simulink model "Droopslx"  (R2021a)
settings: Solver=FixedStepDiscrete  StartTime=0.0  StopTime=0.3  FixedStep=1e-6  RelTol=1e-3
InitFcn:
  | %%Elec
  | Vdc=400;
  | L=1.2e-3;
  | Cf=1e-6;
  | R_Load=20;
  | R1=0.005;
  | 
  | %%PWM
  | f=20000;
  | Ts=1/f;
  | w=314.15926;
  | 
  | %%PID
  | Kpi=30;
  | Kpu=0.1;
  | Kiu=600;
  | 
  | %%下垂控制
  | Ksogi=1;
  | m=0.00038;
  | n=0.001;
  | w_lp=2*pi*25;
  | wref=314.15926;
  | Lv=1e-3;
  | 
  | t1=0.14;
  | t2=0.14;
undefined symbols (not defined in the file): DiscIntNeverNeededParam
libraries: spsSeriesRLCBranchLib x15, spsIGBTDiodeLib x8, simulink x4, spsMultimeterLib x4, spsVoltageMeasurementLib x4, spsBreakerLib x3, spsDCVoltageSourceLib x2, pid_lib x2, spsAlphaBetaZerotodq0Lib x1, spspowerguiLib x1
settings Model: Creator=45276  LastModifiedBy=45276
settings DebuggingCC: UnconnectedInputMsg=none  UnconnectedOutputMsg=none  UnconnectedLineMsg=none

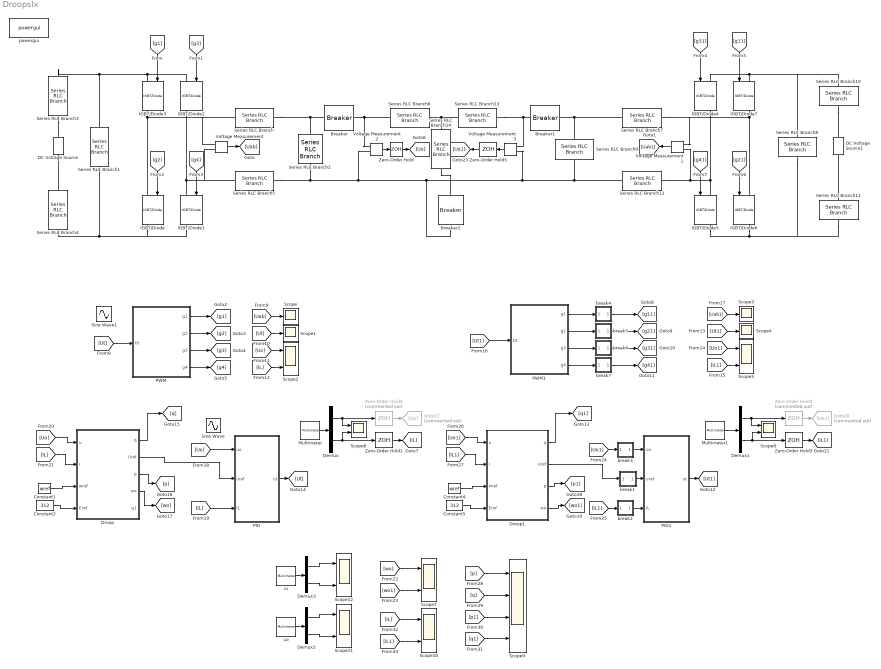
== system Droopslx ==
  Breaker : spsBreakerLib/Breaker  InitialState=0  SwitchingTimes=0  External=off  BreakerResistance=0.0001  SnubberResistance=1e6  SnubberCapacitance=inf  Measurements=None  MoreParameters=on  NoBreakLoop=off
      settings: SourceProductBaseCode=PS
  Breaker1 : spsBreakerLib/Breaker  InitialState=0  SwitchingTimes=t2  External=off  BreakerResistance=0.0001  SnubberResistance=1e6  SnubberCapacitance=inf  Measurements=None  MoreParameters=on  NoBreakLoop=off
      settings: SourceProductBaseCode=PS
  Breaker2 : spsBreakerLib/Breaker  InitialState=0  SwitchingTimes=0.0  External=off  BreakerResistance=0.0001  SnubberResistance=1e6  SnubberCapacitance=inf  Measurements=None  MoreParameters=on  NoBreakLoop=off
      settings: SourceProductBaseCode=PS
  Constant1 : Constant  Value=wref
  Constant2 : Constant  Value=312
  Constant4 : Constant  Value=wref
  Constant5 : Constant  Value=312
  DC Voltage Source : spsDCVoltageSourceLib/DC Voltage Source  Amplitude=Vdc  Measurements=None
  DC Voltage Source1 : spsDCVoltageSourceLib/DC Voltage Source  Amplitude=Vdc  Measurements=None
  Demux{,1..3} (4 alike) : Demux  Outputs=2
  Droop : Subsystem
  Droop1 : Subsystem
  Goto20 : Goto  Commented=on  GotoTag=Uo1
  Goto22 : Goto  Commented=on  GotoTag=Uo
  IGBT/Diode{,1..7} (8 alike) : spsIGBTDiodeLib/IGBT//Diode  Ron=1e-3  Rs=1e5  Cs=inf  Measurements=on
  Multimeter : spsMultimeterLib/Multimeter  PhasorSimulation=off  OutputType=Complex  sel=[1 4]  L=7  Gain=[1 1]  yselected={'Ub: Series RLC Branch2','Ib: Series RLC Branch'};  PSBOutputType=1  PSBequivalent=0  AxesSetting=[0,0.1,-100,100]  Display=0  SavedBlockNames=-11
  Multimeter1 : spsMultimeterLib/Multimeter  PhasorSimulation=off  OutputType=Complex  sel=[3 7]  L=7  Gain=[1 1]  yselected={'Ub: Series RLC Branch9','Ib: Series RLC Branch7'};  PSBOutputType=1  PSBequivalent=0  AxesSetting=[0,0.1,-100,100]  Display=0  SavedBlockNames=-11
  PID : Subsystem
  PID1 : Subsystem
  PWM : Subsystem
  PWM1 : Subsystem
  Scope{,1,3..4} (4 alike) : Scope
  Scope{2,5..8,10..12} (8 alike) : Scope  NumInputPorts=2
  Scope9 : Scope  NumInputPorts=4
  Series RLC Branch : spsSeriesRLCBranchLib/Series RLC Branch  LConnTagsString=__new0  RConnTagsString=__new0  BranchType=RL  Resistance=R1/2  Inductance=L  SetiL0=off  InitialCurrent=0  Capacitance=1e-6  Setx0=off  InitialVoltage=0  Measurements=Branch current
  Series RLC Branch1 : spsSeriesRLCBranchLib/Series RLC Branch  LConnTagsString=__new0  RConnTagsString=__new0  BranchType=C  Resistance=1  Inductance=1e-3  SetiL0=off  InitialCurrent=0  Capacitance=Cf  Setx0=off  InitialVoltage=0  Measurements=None
  Series RLC Branch{3..4,10..11} (4 alike) : spsSeriesRLCBranchLib/Series RLC Branch  LConnTagsString=__new0  RConnTagsString=__new0  BranchType=R  Resistance=R1  Inductance=1e-3  SetiL0=off  InitialCurrent=0  Capacitance=1e-6  Setx0=off  InitialVoltage=0  Measurements=None
  Series RLC Branch12 : spsSeriesRLCBranchLib/Series RLC Branch  LConnTagsString=__new0  RConnTagsString=__new0  BranchType=RL  Resistance=R1/2  Inductance=L  SetiL0=off  InitialCurrent=0  Capacitance=1e-6  Setx0=off  InitialVoltage=0  Measurements=None
  Series RLC Branch13 : spsSeriesRLCBranchLib/Series RLC Branch  LConnTagsString=__new0  RConnTagsString=__new0  BranchType=R  Resistance=0.005  Inductance=1e-3  SetiL0=off  InitialCurrent=0  Capacitance=1e-6  Setx0=off  InitialVoltage=0  Measurements=Branch current
  Series RLC Branch14 : spsSeriesRLCBranchLib/Series RLC Branch  LConnTagsString=__new0  RConnTagsString=__new0  BranchType=R  Resistance=R_Load  Inductance=1e-3  SetiL0=off  InitialCurrent=0  Capacitance=1e-6  Setx0=off  InitialVoltage=0  Measurements=None
  Series RLC Branch2 : spsSeriesRLCBranchLib/Series RLC Branch  LConnTagsString=__new0  RConnTagsString=__new0  BranchType=C  Resistance=1  Inductance=1e-3  SetiL0=off  InitialCurrent=0  Capacitance=Cf  Setx0=off  InitialVoltage=0  Measurements=Branch voltage
  Series RLC Branch5 : spsSeriesRLCBranchLib/Series RLC Branch  LConnTagsString=__new0  RConnTagsString=__new0  BranchType=RL  Resistance=R1/2  Inductance=L  SetiL0=off  InitialCurrent=0  Capacitance=1e-6  Setx0=off  InitialVoltage=0  Measurements=None
  Series RLC Branch6 : spsSeriesRLCBranchLib/Series RLC Branch  LConnTagsString=__new0  RConnTagsString=__new0  BranchType=R  Resistance=0.001  Inductance=1e-3  SetiL0=off  InitialCurrent=0  Capacitance=1e-6  Setx0=off  InitialVoltage=0  Measurements=Branch voltage and current
  Series RLC Branch7 : spsSeriesRLCBranchLib/Series RLC Branch  LConnTagsString=__new0  RConnTagsString=__new0  BranchType=RL  Resistance=R1/2  Inductance=L  SetiL0=off  InitialCurrent=0  Capacitance=1e-6  Setx0=off  InitialVoltage=0  Measurements=Branch current
  Series RLC Branch8 : spsSeriesRLCBranchLib/Series RLC Branch  LConnTagsString=__new0  RConnTagsString=__new0  BranchType=C  Resistance=1  Inductance=1e-3  SetiL0=off  InitialCurrent=0  Capacitance=Cf  Setx0=off  InitialVoltage=0  Measurements=None
  Series RLC Branch9 : spsSeriesRLCBranchLib/Series RLC Branch  LConnTagsString=__new0  RConnTagsString=__new0  BranchType=C  Resistance=1  Inductance=1e-3  SetiL0=off  InitialCurrent=0  Capacitance=Cf  Setx0=off  InitialVoltage=0  Measurements=Branch voltage
  Sine Wave : Sin  Amplitude=400  Frequency=2*pi*50  SampleTime=Ts
  Sine Wave1 : Sin  Frequency=2*pi*50  SampleTime=0
  Voltage Measurement{,1..3} (4 alike) : spsVoltageMeasurementLib/Voltage Measurement  PhasorSimulation=off  OutputType=Complex  PSBequivalent=0
  Zero-Order Hold : ZeroOrderHold  SampleTime=Ts
  Zero-Order Hold1 : ZeroOrderHold  SampleTime=Ts
  Zero-Order Hold2 : ZeroOrderHold  Commented=on  SampleTime=-1
  Zero-Order Hold3 : ZeroOrderHold  SampleTime=-1
  Zero-Order Hold4 : ZeroOrderHold  Commented=on  SampleTime=Ts
  Zero-Order Hold5 : ZeroOrderHold  SampleTime=Ts
  break1 : Subsystem
  break2 : Subsystem
  break3 : Subsystem
  break4 : Subsystem
  break5 : Subsystem
  break6 : Subsystem
  break7 : Subsystem
  io : spsMultimeterLib/Multimeter  PhasorSimulation=off  OutputType=Complex  sel=[6 5]  L=7  Gain=[1 1]  yselected={'Ib: Series RLC Branch6','Ib: Series RLC Branch13'};  PSBOutputType=1  PSBequivalent=0  AxesSetting=[0,0.1,-100,100]  Display=0  SavedBlockNames=-11
  powergui : spspowerguiLib/powergui  Priority=1  SimulationMode=Discrete  SampleTime=1e-6  frequency=60  Iterations=50  frequencyindice=0  Pbase=100e6  ErrMax=1e-4  UnitsV=kV  UnitsW=MW  buscounter=0  FunctionMessages=off  echomessages=off  EnableUseOfTLC=off  CurrentSourceSwitches=off  DisableSnubberDevices=off  DisableRonSwitches=off  DisableVfSwitches=off  DisplayEquations=off  AutomaticDiscreteSolvers=off  SolverType=Tustin/Backward Euler (TBE)  Interpol=off  ExternalGateDelay=off  methode=off  Ts=100  x0status=blocks  SPID=on  SwTol=0  HookPort=off  NonlinearTolerance=1e-4  nMaxIteration=100  ContinueOnMaxIteration=off  RestoreLinks=warning  ResistiveCurrentMeasurement=off  Frange=[0:2:500]  Ylog=off  Xlog=on  ShowGrid=off  save=off  variable=ZData  structure=0  ZoomFFT=off  StartTime=0.0  cycles=1  DisplayStyle=1  fundamental=60  FreqAxis=off  MaxFrequency=1000  frequencyindicesteady=1  RmsSteady=1  display=off
  uo : spsMultimeterLib/Multimeter  PhasorSimulation=off  OutputType=Complex  sel=[1 3]  L=7  Gain=[1 1]  yselected={'Ub: Series RLC Branch2','Ub: Series RLC Branch9'};  PSBOutputType=1  PSBequivalent=0  AxesSetting=[0,0.1,-100,100]  Display=0  SavedBlockNames=-11
  wires:
  Voltage Measurement/1 -> [Uab]
  Voltage Measurement1/1 -> [Uab1]
  [g1] -> IGBT/Diode3/1
  [g3] -> IGBT/Diode2/1
  [g4] -> IGBT/Diode1/1
  [g2] -> IGBT/Diode/1
  [g31] -> IGBT/Diode4/1
  [g11] -> IGBT/Diode7/1
  [g41] -> IGBT/Diode5/1
  [g21] -> IGBT/Diode6/1
  PWM/1(g1) -> [g1]
  PWM/2(g2) -> [g2]
  PWM/3(g3) -> [g3]
  PWM/4(g4) -> [g4]
  [Uab] -> Scope/1
  [Ut] -> Scope1/1
  [Uo] -> Scope2/1
  [IL] -> Scope2/2
  [IL1] -> Scope5/2
  [Uo1] -> Scope5/1
  [Ut1] -> Scope4/1
  [Uab1] -> Scope3/1
  PWM1/1(g1) -> break4/1(in)
  [Ut1] -> PWM1/1(Ut)
  [IL] -> PID/3(IL)
  PID/1(ut) -> [Ut]
  [Uo] -> Droop/1(u)
  Constant1/1 -> Droop/3(wref)
  Constant2/1 -> Droop/4(Eref)
  Droop/1(q) -> [q]
  Droop/3(p) -> [p]
  Droop/4(wo) -> [wo]
  Multimeter/1 -> Demux/1
  Demux/2 -> Scope6/2, Zero-Order Hold1/1
  Demux/1 -> Zero-Order Hold4/1, Scope6/1
  Zero-Order Hold1/1 -> [IL]
  [wo] -> Scope7/1
  [wo1] -> Scope7/2
  Zero-Order Hold3/1 -> [IL1]
  Zero-Order Hold2/1 -> Goto20/1
  Demux1/1 -> Zero-Order Hold2/1, Scope8/1
  Demux1/2 -> Zero-Order Hold3/1, Scope8/2
  Multimeter1/1 -> Demux1/1
  Droop1/4(wo) -> [wo1]
  Droop1/3(p) -> [p1]
  Droop1/1(q) -> [q1]
  Constant5/1 -> Droop1/4(Eref)
  Constant4/1 -> Droop1/3(wref)
  [Uo1] -> Droop1/1(u)
  PID1/1(ut) -> [Ut1]
  [IL1] -> break2/1(in)
  [p] -> Scope9/1
  [q] -> Scope9/2
  [p1] -> Scope9/3
  [q1] -> Scope9/4
  [IL1] -> Droop1/2(I)
  [Uo] -> PID/1(uo)
  [Uo1] -> break3/1(in)
  [Ut] -> PWM/1(Ut)
  Droop/2(Uref) -> PID/2(uref)
  [IL] -> Droop/2(I)
  [IL] -> Scope10/1
  [IL1] -> Scope10/2
  break2/1(out) -> PID1/3(IL)
  break3/1(out) -> PID1/1(uo)
  Droop1/2(Uref) -> break1/1(in)
  break4/1(out) -> [g11]
  PWM1/2(g2) -> break5/1(in)
  break5/1(out) -> [g21]
  PWM1/3(g3) -> break6/1(in)
  break6/1(out) -> [g31]
  PWM1/4(g4) -> break7/1(in)
  break7/1(out) -> [g41]
  Zero-Order Hold/1 -> [Uo]
  Voltage Measurement2/1 -> Zero-Order Hold/1
  Zero-Order Hold4/1 -> Goto22/1
  Zero-Order Hold5/1 -> [Uo1]
  Voltage Measurement3/1 -> Zero-Order Hold5/1
  break1/1(out) -> PID1/2(uref)
  Demux2/1 -> Scope11/1
  Demux2/2 -> Scope11/2
  uo/1 -> Demux2/1
  io/1 -> Demux3/1
  Demux3/1 -> Scope12/1
  Demux3/2 -> Scope12/2
  connections:
  Series RLC Branch4/LConn1 -- DC Voltage Source/LConn1
  Series RLC Branch3/RConn1 -- DC Voltage Source/RConn1
  Series RLC Branch3/LConn1 -- Series RLC Branch1/LConn1 -- IGBT/Diode3/LConn1 -- IGBT/Diode2/LConn1
  Voltage Measurement/LConn1 -- Series RLC Branch/LConn1 -- IGBT/Diode3/RConn1 -- IGBT/Diode/LConn1
  IGBT/Diode1/RConn1 -- IGBT/Diode/RConn1 -- Series RLC Branch1/RConn1 -- Series RLC Branch4/RConn1
  Voltage Measurement/LConn2 -- Series RLC Branch5/LConn1 -- IGBT/Diode2/RConn1 -- IGBT/Diode1/LConn1
  Series RLC Branch/RConn1 -- Breaker/LConn1 -- Series RLC Branch2/LConn1
  Series RLC Branch8/LConn1 -- Series RLC Branch10/LConn1 -- IGBT/Diode7/LConn1 -- IGBT/Diode4/LConn1
  Voltage Measurement1/LConn2 -- Series RLC Branch7/LConn1 -- IGBT/Diode7/RConn1 -- IGBT/Diode6/LConn1
  Series RLC Branch11/RConn1 -- Series RLC Branch8/RConn1 -- IGBT/Diode6/RConn1 -- IGBT/Diode5/RConn1
  Series RLC Branch12/LConn1 -- Voltage Measurement1/LConn1 -- IGBT/Diode5/LConn1 -- IGBT/Diode4/RConn1
  Series RLC Branch7/RConn1 -- Breaker1/RConn1 -- Series RLC Branch9/LConn1
  Series RLC Branch12/RConn1 -- Voltage Measurement3/LConn2 -- Breaker2/LConn1 -- Voltage Measurement2/LConn2 -- Series RLC Branch5/RConn1 -- Series RLC Branch2/RConn1 -- Series RLC Branch9/RConn1
  Series RLC Branch11/LConn1 -- DC Voltage Source1/LConn1
  Series RLC Branch10/RConn1 -- DC Voltage Source1/RConn1
  Series RLC Branch6/LConn1 -- Series RLC Branch14/LConn1 -- Series RLC Branch13/LConn1
  Series RLC Branch13/RConn1 -- Voltage Measurement3/LConn1 -- Breaker1/LConn1
  Breaker/RConn1 -- Voltage Measurement2/LConn1 -- Series RLC Branch6/RConn1
  Series RLC Branch14/RConn1 -- Breaker2/RConn1

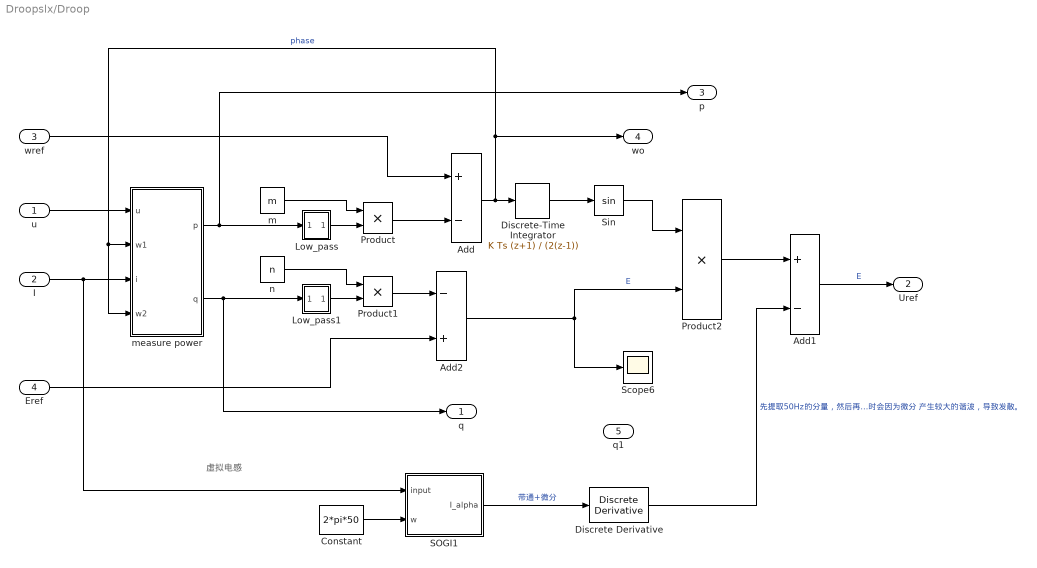
== system Droopslx/Droop ==
  note: 虚拟电感
  u : Inport
  I : Inport  Port=2
  wref : Inport  Port=3
  Eref : Inport  Port=4
  Add : Sum  Inputs=+-
  Add1 : Sum  Inputs=+-
  Add2 : Sum  Inputs=-+
  Constant : Constant  Value=2*pi*50
  Discrete Derivative : simulink/Discrete/Discrete Derivative  gainval=Lv  ICPrevScaledInput=0.0  OutMin=[]  OutMax=[]  OutDataType=fixdt(1, 16)  OutScaling=2^-10  DoSatur=off
  Discrete-Time Integrator : DiscreteIntegrator  IntegratorMethod=Integration: Trapezoidal  SampleTime=Ts  ICPrevOutput=DiscIntNeverNeededParam  ICPrevScaledInput=DiscIntNeverNeededParam
  Low_pass : Subsystem
  Low_pass1 : Subsystem
  Product : Product
  Product1 : Product
  Product2 : Product
  SOGI1 : Subsystem
  Scope6 : Scope
  Sin : Trigonometry
  m : Constant  Value=m
  measure power : Subsystem
  n : Constant  Value=n
  q : Outport
  Uref : Outport  Port=2
  p : Outport  Port=3
  wo : Outport  Port=4
  q1 : Outport  Port=5
  wires:
  measure power/1(p) -> p/1, Low_pass/1(in)
  Add2/1 -> Scope6/1, Product2/2  "E"
  Add/1 -> measure power/4(w2), measure power/2(w1), wo/1, Discrete-Time Integrator/1  "phase"
  measure power/2(q) -> q/1, Low_pass1/1(in)
  Discrete-Time Integrator/1 -> Sin/1
  I/1 -> SOGI1/1(input), measure power/3(i)
  m/1 -> Product/1
  Product2/1 -> Add1/1
  Low_pass/1(out) -> Product/2
  Sin/1 -> Product2/1
  Product1/1 -> Add2/1
  n/1 -> Product1/1
  Eref/1 -> Add2/2
  u/1 -> measure power/1(u)
  Low_pass1/1(out) -> Product1/2
  Add1/1 -> Uref/1  "E"
  Product/1 -> Add/2
  wref/1 -> Add/1
  SOGI1/1(I_alpha) -> Discrete Derivative/1  "带通+微分"
  Constant/1 -> SOGI1/2(w)
  Discrete Derivative/1 -> Add1/2  "先提取50Hz的分量，然后再取微分。 如果先取微分，再用SOGI提取时会因为微分 产生较大的谐波，导致发散。"

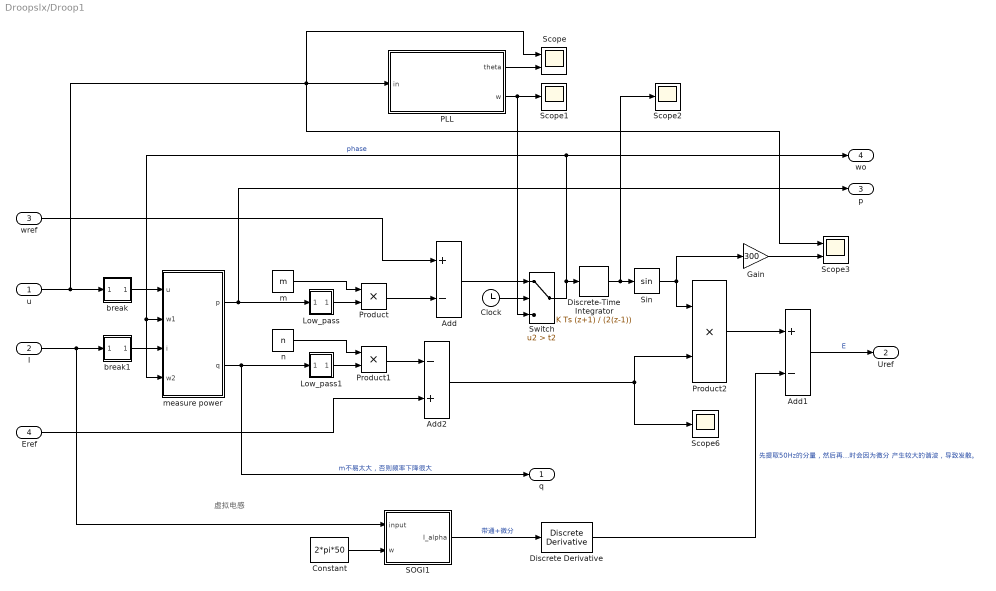
== system Droopslx/Droop1 ==
  note: 虚拟电感
  u : Inport
  I : Inport  Port=2
  wref : Inport  Port=3
  Eref : Inport  Port=4
  Add : Sum  Inputs=+-
  Add1 : Sum  Inputs=+-
  Add2 : Sum  Inputs=-+
  Clock : Clock
  Constant : Constant  Value=2*pi*50
  Discrete Derivative : simulink/Discrete/Discrete Derivative  gainval=Lv  ICPrevScaledInput=0.0  OutMin=[]  OutMax=[]  OutDataType=fixdt(1, 16)  OutScaling=2^-10  DoSatur=off
  Discrete-Time Integrator : DiscreteIntegrator  IntegratorMethod=Integration: Trapezoidal  SampleTime=Ts  ICPrevOutput=DiscIntNeverNeededParam  ICPrevScaledInput=DiscIntNeverNeededParam
  Gain : Gain  Gain=300
  Low_pass : Subsystem
  Low_pass1 : Subsystem
  PLL : Subsystem
  Product : Product
  Product1 : Product
  Product2 : Product
  SOGI1 : Subsystem
  Scope : Scope  NumInputPorts=2
  Scope1 : Scope
  Scope2 : Scope
  Scope3 : Scope  NumInputPorts=2
  Scope6 : Scope
  Sin : Trigonometry
  Switch : Switch  Criteria=u2 > Threshold  Threshold=t2
  break : Subsystem
  break1 : Subsystem
  m : Constant  Value=m
  measure power : Subsystem
  n : Constant  Value=n
  q : Outport
  Uref : Outport  Port=2
  p : Outport  Port=3
  wo : Outport  Port=4
  wires:
  wref/1 -> Add/1
  Product/1 -> Add/2
  Add1/1 -> Uref/1  "E"
  Low_pass1/1(out) -> Product1/2
  u/1 -> break/1(in), Scope3/1, Scope/1, PLL/1(in)
  Eref/1 -> Add2/2
  n/1 -> Product1/1
  Product1/1 -> Add2/1
  Sin/1 -> Product2/1, Gain/1
  Low_pass/1(out) -> Product/2
  Product2/1 -> Add1/1
  m/1 -> Product/1
  I/1 -> SOGI1/1(input), break1/1(in)
  Discrete-Time Integrator/1 -> Scope2/1, Sin/1
  measure power/2(q) -> Low_pass1/1(in), q/1  "m不易太大，否则频率下降很大"
  Add/1 -> Switch/1
  Add2/1 -> Product2/2, Scope6/1
  measure power/1(p) -> Low_pass/1(in), p/1
  Clock/1 -> Switch/2
  Switch/1 -> wo/1, measure power/4(w2), measure power/2(w1), Discrete-Time Integrator/1  "phase"
  Gain/1 -> Scope3/2
  PLL/1(theta) -> Scope/2
  PLL/2(w) -> Switch/3, Scope1/1
  break/1(out) -> measure power/1(u)
  break1/1(out) -> measure power/3(i)
  Constant/1 -> SOGI1/2(w)
  SOGI1/1(I_alpha) -> Discrete Derivative/1  "带通+微分"
  Discrete Derivative/1 -> Add1/2  "先提取50Hz的分量，然后再取微分。 如果先取微分，再用SOGI提取时会因为微分 产生较大的谐波，导致发散。"

== system Droopslx/PID ==
  note: 前馈控制
  note: 电压环
  note: 电流环
  uo : Inport
  uref : Inport  Port=2
  IL : Inport  Port=3
  Gain : Gain  Gain=Kpi
  Gain1 : Gain  Gain=1/400
  PID Controller : pid_lib/PID Controller  Controller=PI  Form=Parallel  TimeDomain=Discrete-time  UseExternalTs=off  SampleTime=Ts  IntegratorMethod=Trapezoidal  FilterMethod=Forward Euler  ControllerParametersSource=internal  P=Kpu  I=Kiu  D=0  UseFilter=on  N=100  TunerSelectOption=Transfer Function Based (PID Tuner App)  InitialConditionSource=internal  InitialConditionForIntegrator=0  InitialConditionForFilter=0  DifferentiatorICPrevScaledInput=0  ExternalReset=none  TrackingMode=off  Kt=1  LimitOutput=off  SatLimitsSource=internal  UpperSaturationLimit=inf  LowerSaturationLimit=-inf  LinearizeAsGain=on  AntiWindupMode=none  Kb=1  POutMin=[]  POutMax=[]  IOutMin=[]  IOutMax=[]  DOutMin=[]  DOutMax=[]  NOutMin=[]  NOutMax=[]  SumOutMin=[]  SumOutMax=[]  SaturationOutMin=[]  SaturationOutMax=[]  PParamMin=[]  PParamMax=[]  IParamMin=[]  IParamMax=[]  DParamMin=[]  DParamMax=[]  NParamMin=[]  NParamMax=[]  KbParamMin=[]  KbParamMax=[]  KtParamMin=[]  KtParamMax=[]  KbOutMin=[]  KbOutMax=[]  KtOutMin=[]  KtOutMax=[]  IntegratorOutMin=[]  IntegratorOutMax=[]  FilterOutMin=[]  FilterOutMax=[]  SumI1OutMin=[]  SumI1OutMax=[]  SumI2OutMin=[]  SumI2OutMax=[]  SumI3OutMin=[]  SumI3OutMax=[]  SumI4OutMin=[]  SumI4OutMax=[]  SumDOutMin=[]  SumDOutMax=[]  DifferentiatorOutMin=[]  DifferentiatorOutMax=[]  FilterDiffOutCoefMin=[]  FilterDiffOutCoefMax=[]  ReciprocalOutMin=[]  ReciprocalOutMax=[]  SumDenOutMin=[]  SumDenOutMax=[]  SumNumOutMin=[]  SumNumOutMax=[]  DivideOutMin=[]  DivideOutMax=[]  UdiffTsProdOutMin=[]  UdiffTsProdOutMax=[]  NTsProdOutMin=[]  NTsProdOutMax=[]  UintegralTsProdOutMin=[]  UintegralTsProdOutMax=[]  UngainTsProdOutMin=[]  UngainTsProdOutMax=[]  IntegratorContinuousStateAttributes=''  IntegratorStateMustResolveToSignalObject=off  IntegratorRTWStateStorageClass=Auto  FilterContinuousStateAttributes=''  FilterStateMustResolveToSignalObject=off  FilterRTWStateStorageClass=Auto  ParallelPVariant=InternalParameters  IdealPVariant=Disabled  IVariant=InternalParameters  DVariant=Disabled  IntegratorVariant=Discrete  SatVariant=Disabled  AWVariant=Passthrough  PCopyVariant=Disabled  TRVariant=Disabled  FdbkBlocksVariant=Forward  IdealPFdbkVariant=Disabled  SatFdbkVariant=Disabled  DerivativeFilterVariant=Disabled  NVariant=Disabled  NCopyVariant=Disabled_SignalSpec  FilterICVariant=Disabled  IntegratorICVariant=InternalICs  ExternalResetVariant=Disabled  TRSumVariant=Passthrough  SumFdbkVariant=Disabled  SumVariant=Sum_PI  TsampFilterVariant=InternalTs  TsampNgainVariant=Passthrough  TsampIntegralVariant=Passthrough  ExternalSaturationOutDataTypeStr=Inherit: Same as second input
  Sum : Sum  Inputs=|+-
  Sum1 : Sum  Inputs=|+-
  Sum2 : Sum  Inputs=|++
  ut : Outport
  wires:
  Gain/1 -> Sum2/1
  PID Controller/1 -> Sum1/1
  Sum1/1 -> Gain/1
  uo/1 -> Sum2/2, Sum/2
  IL/1 -> Sum1/2
  uref/1 -> Sum/1
  Sum/1 -> PID Controller/1
  Sum2/1 -> Gain1/1
  Gain1/1 -> ut/1

== system Droopslx/PID1 ==
  note: 电流环
  note: 电压环
  uo : Inport
  uref : Inport  Port=2
  IL : Inport  Port=3
  Gain : Gain  Gain=Kpi
  Gain1 : Gain  Gain=1/400
  PID Controller : pid_lib/PID Controller  Controller=PI  Form=Parallel  TimeDomain=Discrete-time  UseExternalTs=off  SampleTime=Ts  IntegratorMethod=Trapezoidal  FilterMethod=Forward Euler  ControllerParametersSource=internal  P=Kpu  I=Kiu  D=0  UseFilter=on  N=100  TunerSelectOption=Transfer Function Based (PID Tuner App)  InitialConditionSource=internal  InitialConditionForIntegrator=0  InitialConditionForFilter=0  DifferentiatorICPrevScaledInput=0  ExternalReset=none  TrackingMode=off  Kt=1  LimitOutput=off  SatLimitsSource=internal  UpperSaturationLimit=inf  LowerSaturationLimit=-inf  LinearizeAsGain=on  AntiWindupMode=none  Kb=1  POutMin=[]  POutMax=[]  IOutMin=[]  IOutMax=[]  DOutMin=[]  DOutMax=[]  NOutMin=[]  NOutMax=[]  SumOutMin=[]  SumOutMax=[]  SaturationOutMin=[]  SaturationOutMax=[]  PParamMin=[]  PParamMax=[]  IParamMin=[]  IParamMax=[]  DParamMin=[]  DParamMax=[]  NParamMin=[]  NParamMax=[]  KbParamMin=[]  KbParamMax=[]  KtParamMin=[]  KtParamMax=[]  KbOutMin=[]  KbOutMax=[]  KtOutMin=[]  KtOutMax=[]  IntegratorOutMin=[]  IntegratorOutMax=[]  FilterOutMin=[]  FilterOutMax=[]  SumI1OutMin=[]  SumI1OutMax=[]  SumI2OutMin=[]  SumI2OutMax=[]  SumI3OutMin=[]  SumI3OutMax=[]  SumI4OutMin=[]  SumI4OutMax=[]  SumDOutMin=[]  SumDOutMax=[]  DifferentiatorOutMin=[]  DifferentiatorOutMax=[]  FilterDiffOutCoefMin=[]  FilterDiffOutCoefMax=[]  ReciprocalOutMin=[]  ReciprocalOutMax=[]  SumDenOutMin=[]  SumDenOutMax=[]  SumNumOutMin=[]  SumNumOutMax=[]  DivideOutMin=[]  DivideOutMax=[]  UdiffTsProdOutMin=[]  UdiffTsProdOutMax=[]  NTsProdOutMin=[]  NTsProdOutMax=[]  UintegralTsProdOutMin=[]  UintegralTsProdOutMax=[]  UngainTsProdOutMin=[]  UngainTsProdOutMax=[]  IntegratorContinuousStateAttributes=''  IntegratorStateMustResolveToSignalObject=off  IntegratorRTWStateStorageClass=Auto  FilterContinuousStateAttributes=''  FilterStateMustResolveToSignalObject=off  FilterRTWStateStorageClass=Auto  ParallelPVariant=InternalParameters  IdealPVariant=Disabled  IVariant=InternalParameters  DVariant=Disabled  IntegratorVariant=Discrete  SatVariant=Disabled  AWVariant=Passthrough  PCopyVariant=Disabled  TRVariant=Disabled  FdbkBlocksVariant=Forward  IdealPFdbkVariant=Disabled  SatFdbkVariant=Disabled  DerivativeFilterVariant=Disabled  NVariant=Disabled  NCopyVariant=Disabled_SignalSpec  FilterICVariant=Disabled  IntegratorICVariant=InternalICs  ExternalResetVariant=Disabled  TRSumVariant=Passthrough  SumFdbkVariant=Disabled  SumVariant=Sum_PI  TsampFilterVariant=InternalTs  TsampNgainVariant=Passthrough  TsampIntegralVariant=Passthrough  ExternalSaturationOutDataTypeStr=Inherit: Same as second input
  Sum : Sum  Inputs=|+-
  Sum1 : Sum  Inputs=|+-
  Sum2 : Sum  Inputs=|++
  ut : Outport
  wires:
  Gain1/1 -> ut/1
  Sum2/1 -> Gain1/1
  Sum/1 -> PID Controller/1
  uref/1 -> Sum/1
  IL/1 -> Sum1/2
  uo/1 -> Sum/2, Sum2/2
  Sum1/1 -> Gain/1
  PID Controller/1 -> Sum1/1
  Gain/1 -> Sum2/1

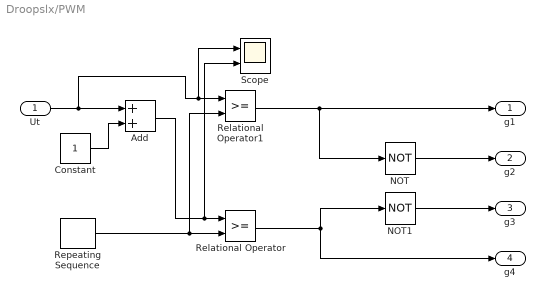
== system Droopslx/PWM ==
  Ut : Inport
  Add : Sum
  Constant : Constant
  NOT : Logic  Operator=NOT  IconShape=distinctive  AllPortsSameDT=off  OutDataTypeStr=boolean
  NOT1 : Logic  Operator=NOT  IconShape=distinctive  AllPortsSameDT=off  OutDataTypeStr=boolean
  Relational Operator : RelationalOperator  OutDataTypeStr=boolean  RndMeth=Simplest
  Relational Operator1 : RelationalOperator  OutDataTypeStr=boolean  RndMeth=Simplest
  Repeating Sequence : simulink/Sources/Repeating Sequence  rep_seq_t=[0 Ts/2 Ts]  rep_seq_y=[0 1 0]
  Scope : Scope  NumInputPorts=2
  g1 : Outport
  g2 : Outport  Port=2
  g3 : Outport  Port=3
  g4 : Outport  Port=4
  wires:
  Add/1 -> Scope/2, Relational Operator/1
  Constant/1 -> Add/2
  Relational Operator1/1 -> g1/1, NOT/1
  Relational Operator/1 -> g4/1, NOT1/1
  NOT/1 -> g2/1
  Ut/1 -> Scope/1, Relational Operator1/1, Add/1
  NOT1/1 -> g3/1
  Repeating Sequence/1 -> Relational Operator1/2, Relational Operator/2

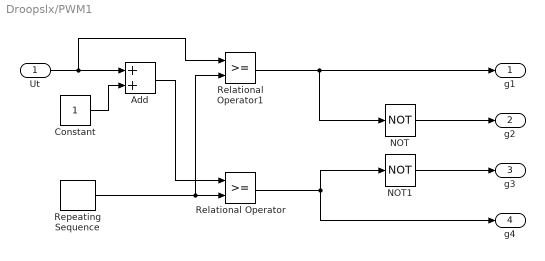
== system Droopslx/PWM1 ==
  Ut : Inport
  Add : Sum
  Constant : Constant
  NOT : Logic  Operator=NOT  IconShape=distinctive  AllPortsSameDT=off  OutDataTypeStr=boolean
  NOT1 : Logic  Operator=NOT  IconShape=distinctive  AllPortsSameDT=off  OutDataTypeStr=boolean
  Relational Operator : RelationalOperator  OutDataTypeStr=boolean  RndMeth=Simplest
  Relational Operator1 : RelationalOperator  OutDataTypeStr=boolean  RndMeth=Simplest
  Repeating Sequence : simulink/Sources/Repeating Sequence  rep_seq_t=[0 Ts/2 Ts]  rep_seq_y=[0 1 0]
  g1 : Outport
  g2 : Outport  Port=2
  g3 : Outport  Port=3
  g4 : Outport  Port=4
  wires:
  NOT1/1 -> g3/1
  Ut/1 -> Add/1, Relational Operator1/1
  NOT/1 -> g2/1
  Relational Operator/1 -> NOT1/1, g4/1
  Relational Operator1/1 -> NOT/1, g1/1
  Constant/1 -> Add/2
  Add/1 -> Relational Operator/1
  Repeating Sequence/1 -> Relational Operator/2, Relational Operator1/2

== system Droopslx/break1 ==
  in : Inport
  Product3 : Product
  Step : Step  Time=t1  SampleTime=0
  out : Outport
  wires:
  Product3/1 -> out/1
  in/1 -> Product3/2
  Step/1 -> Product3/1

== system Droopslx/break2 ==
  in : Inport
  Product3 : Product
  Step : Step  Time=t1  SampleTime=0
  out : Outport
  wires:
  Product3/1 -> out/1
  in/1 -> Product3/2
  Step/1 -> Product3/1

== system Droopslx/break3 ==
  in : Inport
  Product3 : Product
  Step : Step  Time=t1  SampleTime=0
  out : Outport
  wires:
  Product3/1 -> out/1
  in/1 -> Product3/2
  Step/1 -> Product3/1

== system Droopslx/break4 ==
  in : Inport
  Product3 : Product
  Step : Step  Time=t1  SampleTime=0
  out : Outport
  wires:
  Step/1 -> Product3/1
  in/1 -> Product3/2
  Product3/1 -> out/1

== system Droopslx/break5 ==
  in : Inport
  Product3 : Product
  Step : Step  Time=t1  SampleTime=0
  out : Outport
  wires:
  Product3/1 -> out/1
  in/1 -> Product3/2
  Step/1 -> Product3/1

== system Droopslx/break6 ==
  in : Inport
  Product3 : Product
  Step : Step  Time=t1  SampleTime=0
  out : Outport
  wires:
  Product3/1 -> out/1
  in/1 -> Product3/2
  Step/1 -> Product3/1

== system Droopslx/break7 ==
  in : Inport
  Product3 : Product
  Step : Step  Time=t1  SampleTime=0
  out : Outport
  wires:
  Step/1 -> Product3/1
  in/1 -> Product3/2
  Product3/1 -> out/1

== system Droopslx/Droop/Low_pass ==
  in : Inport
  Discrete-Time Integrator : DiscreteIntegrator  IntegratorMethod=Integration: Trapezoidal  gainval=w_lp  SampleTime=Ts  ICPrevOutput=DiscIntNeverNeededParam  ICPrevScaledInput=DiscIntNeverNeededParam
  Sum : Sum  Inputs=|+-
  out : Outport
  wires:
  Sum/1 -> Discrete-Time Integrator/1
  Discrete-Time Integrator/1 -> out/1, Sum/2
  in/1 -> Sum/1

== system Droopslx/Droop/Low_pass1 ==
  in : Inport
  Discrete-Time Integrator : DiscreteIntegrator  IntegratorMethod=Integration: Trapezoidal  gainval=w_lp  SampleTime=Ts  ICPrevOutput=DiscIntNeverNeededParam  ICPrevScaledInput=DiscIntNeverNeededParam
  Sum : Sum  Inputs=|+-
  out : Outport
  wires:
  in/1 -> Sum/1
  Discrete-Time Integrator/1 -> Sum/2, out/1
  Sum/1 -> Discrete-Time Integrator/1

== system Droopslx/Droop/SOGI1 ==
  input : Inport
  w : Inport  Port=2
  Discrete-Time Integrator : DiscreteIntegrator  IntegratorMethod=Integration: Trapezoidal  SampleTime=Ts  ICPrevOutput=DiscIntNeverNeededParam  ICPrevScaledInput=DiscIntNeverNeededParam
  Discrete-Time Integrator1 : DiscreteIntegrator  IntegratorMethod=Integration: Trapezoidal  SampleTime=Ts  ICPrevOutput=DiscIntNeverNeededParam  ICPrevScaledInput=DiscIntNeverNeededParam
  Gain : Gain  Gain=Ksogi
  Product1 : Product
  Product2 : Product
  Sum : Sum  Inputs=-+|
  Sum1 : Sum  Inputs=|+-
  I_alpha : Outport
  wires:
  Sum1/1 -> Discrete-Time Integrator/1
  w/1 -> Product1/2, Product2/1
  Discrete-Time Integrator1/1 -> Product2/2
  Product2/1 -> Sum1/2  "bate"
  Product1/1 -> I_alpha/1, Sum/1, Discrete-Time Integrator1/1  "alpha"
  input/1 -> Sum/2
  Sum/1 -> Gain/1
  Gain/1 -> Sum1/1
  Discrete-Time Integrator/1 -> Product1/1

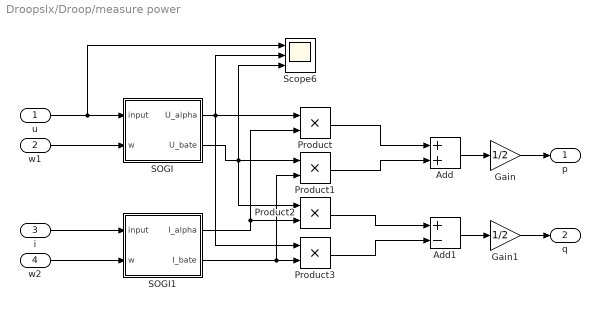
== system Droopslx/Droop/measure power ==
  u : Inport
  w1 : Inport  Port=2
  i : Inport  Port=3
  w2 : Inport  Port=4
  Add : Sum
  Add1 : Sum  Inputs=+-
  Gain : Gain  Gain=1/2
  Gain1 : Gain  Gain=1/2
  Product{,1..3} (4 alike) : Product
  SOGI : Subsystem
  SOGI1 : Subsystem
  Scope6 : Scope  NumInputPorts=3
  p : Outport
  q : Outport  Port=2
  wires:
  w2/1 -> SOGI1/2(w)
  SOGI/2(U_bate) -> Scope6/3, Product2/1, Product1/1
  SOGI1/1(I_alpha) -> Product2/2, Product/2
  w1/1 -> SOGI/2(w)
  u/1 -> Scope6/1, SOGI/1(input)
  Product2/1 -> Add1/1
  Product1/1 -> Add/2
  SOGI/1(U_alpha) -> Scope6/2, Product3/1, Product/1
  Product/1 -> Add/1
  Product3/1 -> Add1/2
  SOGI1/2(I_bate) -> Product3/2, Product1/2
  Add1/1 -> Gain1/1
  i/1 -> SOGI1/1(input)
  Add/1 -> Gain/1
  Gain/1 -> p/1
  Gain1/1 -> q/1

== system Droopslx/Droop1/Low_pass ==
  in : Inport
  Discrete-Time Integrator : DiscreteIntegrator  IntegratorMethod=Integration: Trapezoidal  gainval=w_lp  SampleTime=Ts  ICPrevOutput=DiscIntNeverNeededParam  ICPrevScaledInput=DiscIntNeverNeededParam
  Sum : Sum  Inputs=|+-
  out : Outport
  wires:
  in/1 -> Sum/1
  Discrete-Time Integrator/1 -> Sum/2, out/1
  Sum/1 -> Discrete-Time Integrator/1

== system Droopslx/Droop1/Low_pass1 ==
  in : Inport
  Discrete-Time Integrator : DiscreteIntegrator  IntegratorMethod=Integration: Trapezoidal  gainval=w_lp  SampleTime=Ts  ICPrevOutput=DiscIntNeverNeededParam  ICPrevScaledInput=DiscIntNeverNeededParam
  Sum : Sum  Inputs=|+-
  out : Outport
  wires:
  Sum/1 -> Discrete-Time Integrator/1
  Discrete-Time Integrator/1 -> out/1, Sum/2
  in/1 -> Sum/1

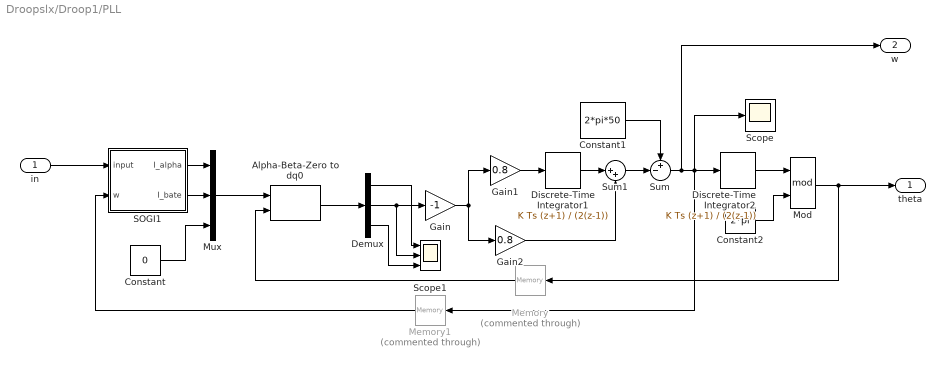
== system Droopslx/Droop1/PLL ==
  in : Inport
  Alpha-Beta-Zero to dq0 : spsAlphaBetaZerotodq0Lib/Alpha-Beta-Zero to dq0  Alignment=90 degrees behind phase A axis
      settings: SourceProductBaseCode=PS
  Constant : Constant  Value=0
  Constant1 : Constant  Value=2*pi*50
  Constant2 : Constant  Value=2*pi
  Demux : Demux  Outputs=3
  Discrete-Time Integrator1 : DiscreteIntegrator  IntegratorMethod=Integration: Trapezoidal  SampleTime=Ts  ICPrevOutput=DiscIntNeverNeededParam  ICPrevScaledInput=DiscIntNeverNeededParam
  Discrete-Time Integrator2 : DiscreteIntegrator  IntegratorMethod=Integration: Trapezoidal  SampleTime=Ts  ICPrevOutput=DiscIntNeverNeededParam  ICPrevScaledInput=DiscIntNeverNeededParam
  Gain : Gain  Gain=-1
  Gain1 : Gain  Gain=0.8
  Gain2 : Gain  Gain=0.8
  Memory : Memory  Commented=through
  Memory1 : Memory  Commented=through
  Mod : Math  Operator=mod  SaturateOnIntegerOverflow=on
  Mux : Mux  Inputs=3
  SOGI1 : Subsystem
  Scope : Scope
  Scope1 : Scope  NumInputPorts=3
  Sum : Sum  Inputs=+-|
  Sum1 : Sum  Inputs=|++
  theta : Outport
  w : Outport  Port=2
  wires:
  Demux/2 -> Gain/1, Scope1/2
  Sum/1 -> w/1, Memory1/1, Scope/1, Discrete-Time Integrator2/1
  Gain2/1 -> Sum1/2
  Alpha-Beta-Zero to dq0/1 -> Demux/1
  Mod/1 -> theta/1, Memory/1
  Discrete-Time Integrator1/1 -> Sum1/1
  Gain/1 -> Gain2/1, Gain1/1
  Mux/1 -> Alpha-Beta-Zero to dq0/1
  Discrete-Time Integrator2/1 -> Mod/1
  SOGI1/2(I_bate) -> Mux/2
  Memory/1 -> Alpha-Beta-Zero to dq0/2
  Constant2/1 -> Mod/2
  in/1 -> SOGI1/1(input)
  Memory1/1 -> SOGI1/2(w)
  Sum1/1 -> Sum/2
  SOGI1/1(I_alpha) -> Mux/1
  Constant1/1 -> Sum/1
  Gain1/1 -> Discrete-Time Integrator1/1
  Constant/1 -> Mux/3
  Demux/3 -> Scope1/3
  Demux/1 -> Scope1/1

== system Droopslx/Droop1/SOGI1 ==
  input : Inport
  w : Inport  Port=2
  Discrete-Time Integrator : DiscreteIntegrator  IntegratorMethod=Integration: Trapezoidal  SampleTime=Ts  ICPrevOutput=DiscIntNeverNeededParam  ICPrevScaledInput=DiscIntNeverNeededParam
  Discrete-Time Integrator1 : DiscreteIntegrator  IntegratorMethod=Integration: Trapezoidal  SampleTime=Ts  ICPrevOutput=DiscIntNeverNeededParam  ICPrevScaledInput=DiscIntNeverNeededParam
  Gain : Gain  Gain=Ksogi
  Product1 : Product
  Product2 : Product
  Sum : Sum  Inputs=-+|
  Sum1 : Sum  Inputs=|+-
  I_alpha : Outport
  wires:
  Sum1/1 -> Discrete-Time Integrator/1
  w/1 -> Product1/2, Product2/1
  Discrete-Time Integrator1/1 -> Product2/2
  Product2/1 -> Sum1/2  "bate"
  Product1/1 -> I_alpha/1, Sum/1, Discrete-Time Integrator1/1  "alpha"
  input/1 -> Sum/2
  Sum/1 -> Gain/1
  Gain/1 -> Sum1/1
  Discrete-Time Integrator/1 -> Product1/1

== system Droopslx/Droop1/break ==
  in : Inport
  Product3 : Product
  Step : Step  Time=t1  SampleTime=0
  out : Outport
  wires:
  Step/1 -> Product3/1
  in/1 -> Product3/2
  Product3/1 -> out/1

== system Droopslx/Droop1/break1 ==
  in : Inport
  Product3 : Product
  Step : Step  Time=t1  SampleTime=0
  out : Outport
  wires:
  Product3/1 -> out/1
  in/1 -> Product3/2
  Step/1 -> Product3/1

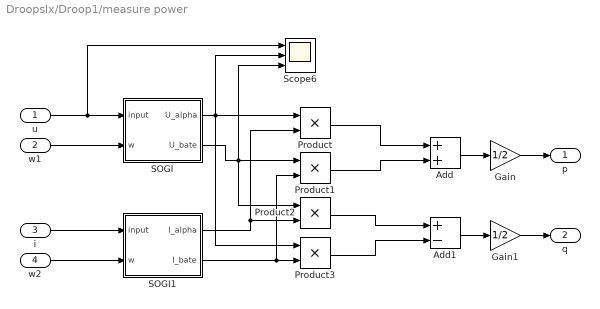
== system Droopslx/Droop1/measure power ==
  u : Inport
  w1 : Inport  Port=2
  i : Inport  Port=3
  w2 : Inport  Port=4
  Add : Sum
  Add1 : Sum  Inputs=+-
  Gain : Gain  Gain=1/2
  Gain1 : Gain  Gain=1/2
  Product{,1..3} (4 alike) : Product
  SOGI : Subsystem
  SOGI1 : Subsystem
  Scope6 : Scope  NumInputPorts=3
  p : Outport
  q : Outport  Port=2
  wires:
  Add/1 -> Gain/1
  i/1 -> SOGI1/1(input)
  Add1/1 -> Gain1/1
  SOGI1/2(I_bate) -> Product1/2, Product3/2
  Product3/1 -> Add1/2
  Product/1 -> Add/1
  SOGI/1(U_alpha) -> Product/1, Product3/1, Scope6/2
  Product1/1 -> Add/2
  Product2/1 -> Add1/1
  u/1 -> SOGI/1(input), Scope6/1
  w1/1 -> SOGI/2(w)
  SOGI1/1(I_alpha) -> Product/2, Product2/2
  SOGI/2(U_bate) -> Product1/1, Product2/1, Scope6/3
  w2/1 -> SOGI1/2(w)
  Gain/1 -> p/1
  Gain1/1 -> q/1

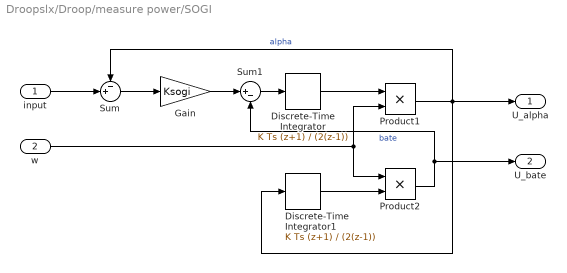
== system Droopslx/Droop/measure power/SOGI ==
  input : Inport
  w : Inport  Port=2
  Discrete-Time Integrator : DiscreteIntegrator  IntegratorMethod=Integration: Trapezoidal  SampleTime=Ts  ICPrevOutput=DiscIntNeverNeededParam  ICPrevScaledInput=DiscIntNeverNeededParam
  Discrete-Time Integrator1 : DiscreteIntegrator  IntegratorMethod=Integration: Trapezoidal  SampleTime=Ts  ICPrevOutput=DiscIntNeverNeededParam  ICPrevScaledInput=DiscIntNeverNeededParam
  Gain : Gain  Gain=Ksogi
  Product1 : Product
  Product2 : Product
  Sum : Sum  Inputs=-+|
  Sum1 : Sum  Inputs=|+-
  U_alpha : Outport
  U_bate : Outport  Port=2
  wires:
  Sum1/1 -> Discrete-Time Integrator/1
  w/1 -> Product1/2, Product2/1
  Discrete-Time Integrator1/1 -> Product2/2
  Product2/1 -> U_bate/1, Sum1/2  "bate"
  Product1/1 -> U_alpha/1, Sum/1, Discrete-Time Integrator1/1  "alpha"
  input/1 -> Sum/2
  Sum/1 -> Gain/1
  Gain/1 -> Sum1/1
  Discrete-Time Integrator/1 -> Product1/1

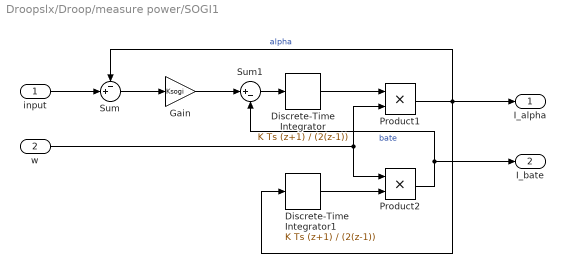
== system Droopslx/Droop/measure power/SOGI1 ==
  input : Inport
  w : Inport  Port=2
  Discrete-Time Integrator : DiscreteIntegrator  IntegratorMethod=Integration: Trapezoidal  SampleTime=Ts  ICPrevOutput=DiscIntNeverNeededParam  ICPrevScaledInput=DiscIntNeverNeededParam
  Discrete-Time Integrator1 : DiscreteIntegrator  IntegratorMethod=Integration: Trapezoidal  SampleTime=Ts  ICPrevOutput=DiscIntNeverNeededParam  ICPrevScaledInput=DiscIntNeverNeededParam
  Gain : Gain  Gain=Ksogi
  Product1 : Product
  Product2 : Product
  Sum : Sum  Inputs=-+|
  Sum1 : Sum  Inputs=|+-
  I_alpha : Outport
  I_bate : Outport  Port=2
  wires:
  Discrete-Time Integrator/1 -> Product1/1
  Gain/1 -> Sum1/1
  Sum/1 -> Gain/1
  input/1 -> Sum/2
  Product1/1 -> Discrete-Time Integrator1/1, Sum/1, I_alpha/1  "alpha"
  Product2/1 -> Sum1/2, I_bate/1  "bate"
  Discrete-Time Integrator1/1 -> Product2/2
  w/1 -> Product2/1, Product1/2
  Sum1/1 -> Discrete-Time Integrator/1

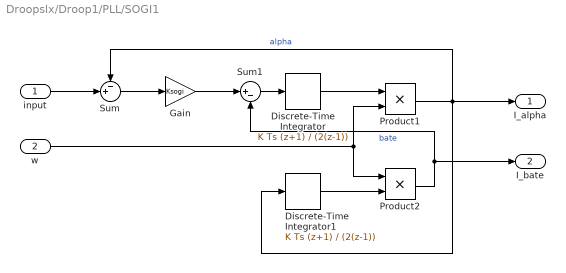
== system Droopslx/Droop1/PLL/SOGI1 ==
  input : Inport
  w : Inport  Port=2
  Discrete-Time Integrator : DiscreteIntegrator  IntegratorMethod=Integration: Trapezoidal  SampleTime=Ts  ICPrevOutput=DiscIntNeverNeededParam  ICPrevScaledInput=DiscIntNeverNeededParam
  Discrete-Time Integrator1 : DiscreteIntegrator  IntegratorMethod=Integration: Trapezoidal  SampleTime=Ts  ICPrevOutput=DiscIntNeverNeededParam  ICPrevScaledInput=DiscIntNeverNeededParam
  Gain : Gain  Gain=Ksogi
  Product1 : Product
  Product2 : Product
  Sum : Sum  Inputs=-+|
  Sum1 : Sum  Inputs=|+-
  I_alpha : Outport
  I_bate : Outport  Port=2
  wires:
  Sum1/1 -> Discrete-Time Integrator/1
  w/1 -> Product1/2, Product2/1
  Discrete-Time Integrator1/1 -> Product2/2
  Product2/1 -> I_bate/1, Sum1/2  "bate"
  Product1/1 -> I_alpha/1, Sum/1, Discrete-Time Integrator1/1  "alpha"
  input/1 -> Sum/2
  Sum/1 -> Gain/1
  Gain/1 -> Sum1/1
  Discrete-Time Integrator/1 -> Product1/1

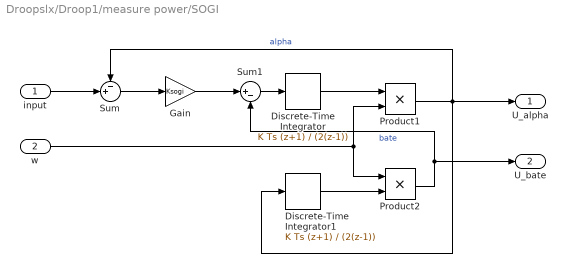
== system Droopslx/Droop1/measure power/SOGI ==
  input : Inport
  w : Inport  Port=2
  Discrete-Time Integrator : DiscreteIntegrator  IntegratorMethod=Integration: Trapezoidal  SampleTime=Ts  ICPrevOutput=DiscIntNeverNeededParam  ICPrevScaledInput=DiscIntNeverNeededParam
  Discrete-Time Integrator1 : DiscreteIntegrator  IntegratorMethod=Integration: Trapezoidal  SampleTime=Ts  ICPrevOutput=DiscIntNeverNeededParam  ICPrevScaledInput=DiscIntNeverNeededParam
  Gain : Gain  Gain=Ksogi
  Product1 : Product
  Product2 : Product
  Sum : Sum  Inputs=-+|
  Sum1 : Sum  Inputs=|+-
  U_alpha : Outport
  U_bate : Outport  Port=2
  wires:
  Discrete-Time Integrator/1 -> Product1/1
  Gain/1 -> Sum1/1
  Sum/1 -> Gain/1
  input/1 -> Sum/2
  Product1/1 -> Discrete-Time Integrator1/1, Sum/1, U_alpha/1  "alpha"
  Product2/1 -> Sum1/2, U_bate/1  "bate"
  Discrete-Time Integrator1/1 -> Product2/2
  w/1 -> Product2/1, Product1/2
  Sum1/1 -> Discrete-Time Integrator/1

== system Droopslx/Droop1/measure power/SOGI1 ==
  input : Inport
  w : Inport  Port=2
  Discrete-Time Integrator : DiscreteIntegrator  IntegratorMethod=Integration: Trapezoidal  SampleTime=Ts  ICPrevOutput=DiscIntNeverNeededParam  ICPrevScaledInput=DiscIntNeverNeededParam
  Discrete-Time Integrator1 : DiscreteIntegrator  IntegratorMethod=Integration: Trapezoidal  SampleTime=Ts  ICPrevOutput=DiscIntNeverNeededParam  ICPrevScaledInput=DiscIntNeverNeededParam
  Gain : Gain  Gain=Ksogi
  Product1 : Product
  Product2 : Product
  Sum : Sum  Inputs=-+|
  Sum1 : Sum  Inputs=|+-
  I_alpha : Outport
  I_bate : Outport  Port=2
  wires:
  Sum1/1 -> Discrete-Time Integrator/1
  w/1 -> Product1/2, Product2/1
  Discrete-Time Integrator1/1 -> Product2/2
  Product2/1 -> I_bate/1, Sum1/2  "bate"
  Product1/1 -> I_alpha/1, Sum/1, Discrete-Time Integrator1/1  "alpha"
  input/1 -> Sum/2
  Sum/1 -> Gain/1
  Gain/1 -> Sum1/1
  Discrete-Time Integrator/1 -> Product1/1
